simulink model "DataCenterStability"  (R2025b)
settings: Solver=daessc  StartTime=0  StopTime=7  FixedStep=5e-5  MaxStep=0.001  RelTol=1e-3
PostLoadFcn:
  | DataCenterParamScan
InitFcn:
  | opFile_ = fullfile(fileparts(which('DataCenterStability')), 'DataCenterStability_SteadyStateOP.mat');
  | if isfile(opFile_)
  |     tmp_ = load(opFile_, 'op');
  |     assignin('base', 'ssOP__', tmp_.op);
  | end
  | warning('off','physmod:common:mf:system:xform:DelayUnsupportedWithOperatingPoint');
  | warning('off','physmod:common:mf:system:xform:TimeUnsupportedWithOperatingPoint');
values from neighbouring files (symbols this model uses):
  baseVoltageDC = ups.Vdc    [DataCenterParamScan.m]
  bessConverterEfficiency = ups.DCBus.converterEff    [DataCenterParamScan.m]
  droopGain = ups.DCBus.droop    [DataCenterParamScan.m]
  filterInductance = ups.inverter.filterInductance    [DataCenterParamScan.m]
  filterInductanceAFE = ups.AFE.filterInductance    [DataCenterParamScan.m]
  filterResistance = ups.inverter.filterResistance    [DataCenterParamScan.m]
  filterResistanceAFE = ups.AFE.filterResistance    [DataCenterParamScan.m]
  frequency = ups.frequency    [DataCenterParamScan.m]
  G1 = 1    [DataCenterParamScan.m]
  G2 = 0    [DataCenterParamScan.m]
  iBatt = ups.batt.iRated    [DataCenterParamScan.m]
  initialMode = ups.batt.initialMode    [DataCenterParamScan.m]
  invKiId = ups.inverter.kiId    [DataCenterParamScan.m]
  invKiVd = ups.inverter.kiVd    [DataCenterParamScan.m]
  invKpId = ups.inverter.kpId    [DataCenterParamScan.m]
  invKpVd = ups.inverter.kpVd    [DataCenterParamScan.m]
  kpDC = ups.DCBus.kpDC    [DataCenterParamScan.m]
  N_pfc = round(N_total * [1/3, 1/3, 1/3])    [DataCenterParamScan.m]    (also in StabilityStudy.m = cfg.Topology.N_pfc)
  plantRating = ups.rating    [DataCenterParamScan.m]
  powerTau = 0.005    [DataCenterParamScan.m]
  rampRate = ups.batt.rampRate    [DataCenterParamScan.m]
  scan = obj.Cfg.GNC    [GNCAnalyzer.m]
  Ts = 5e-5    (= 5e-05)    [DataCenterParamScan.m]
  Vac = ups.Vac    [DataCenterParamScan.m]
  vBattMax = ups.batt.VMax    [DataCenterParamScan.m]
  vBattNom = ups.batt.Vnom    [DataCenterParamScan.m]
  vDCThreshold = ups.DCBus.VThreshold    [DataCenterParamScan.m]
  vGridMin = ups.DCBus.gridThreshold    [DataCenterParamScan.m]
undefined symbols (not defined in the file or in its folder): ctLimitDelayTime, DiscIntNeverNeededParam, ee_sli_rtmsupport, gcbh, itTray, pfc, serverTray, ups
libraries: fl_lib x77, nesl_utility x35, ee_lib x30, simulink x17, eeGeneralControl x14, datacenter_lib x12, eeTransforms x7, slpidlib x4, nesl_utility_internal x4, simulink_extras x3, datacenterCompositeLib x2, eePowerMeasurement x2
(part 5 of 5)

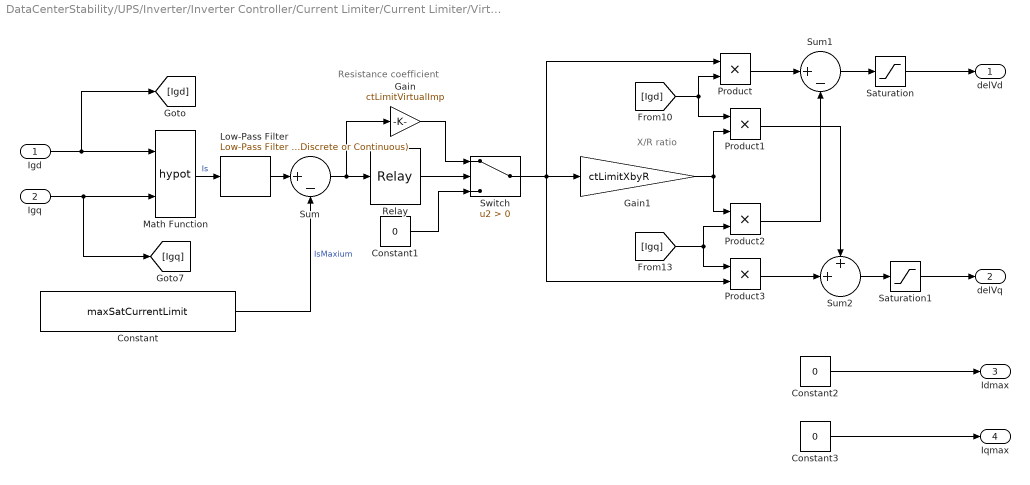
== system DataCenterStability/UPS/Inverter/Inverter Controller/Current Limiter/Current Limiter/Virtual Impedance ==
  note: X/R ratio
  note: Resistance coefficient
  Igd : Inport
  Igq : Inport  Port=2
  Constant : Constant  Value=maxSatCurrentLimit
  Constant1 : Constant  Value=0
  Constant2 : Constant  Value=0
  Constant3 : Constant  Value=0
  Gain : Gain  Gain=ctLimitVirtualImp
  Gain1 : Gain  Gain=ctLimitXbyR
  Low-Pass Filter : eeGeneralControl/Low-Pass Filter (Discrete or Continuous)  K=1  T=1e-3  B=inf  A=-inf  init_option=Inherited from block input  x0=0  Ts=-1
  Math Function : Math  Operator=hypot
  Product{,1..3} (4 alike) : Product
  Relay : Relay  OnSwitchValue=0.01  OffSwitchValue=-0.05
  Saturation : Saturate  UpperLimit=1  LowerLimit=-1
  Saturation1 : Saturate  UpperLimit=1  LowerLimit=-1
  Sum : Sum  Inputs=|+-
  Sum1 : Sum  Inputs=|+-
  Sum2 : Sum  Inputs=++|
  Switch : Switch  Criteria=u2 > Threshold  SaturateOnIntegerOverflow=off  InputSameDT=off
  delVd : Outport
  delVq : Outport  Port=2
  Idmax : Outport  Port=3
  Iqmax : Outport  Port=4
  wires:
  Sum/1 -> Gain/1, Relay/1
  Igq/1 -> [Igq], Math Function/2
  Product1/1 -> Sum2/1
  Gain1/1 -> Product1/2, Product2/1
  Sum1/1 -> Saturation/1
  Product/1 -> Sum1/1
  Product2/1 -> Sum1/2
  Constant/1 -> Sum/2  "IsMaxium"
  Math Function/1 -> Low-Pass Filter/1  "Is"
  [Igq] -> Product3/1, Product2/2
  Switch/1 -> Gain1/1, Product3/2, Product/1
  [Igd] -> Product1/1, Product/2
  Constant2/1 -> Idmax/1
  Constant3/1 -> Iqmax/1
  Gain/1 -> Switch/1
  Constant1/1 -> Switch/3
  Igd/1 -> Math Function/1, [Igd]
  Saturation1/1 -> delVq/1
  Relay/1 -> Switch/2
  Saturation/1 -> delVd/1
  Low-Pass Filter/1 -> Sum/1
  Product3/1 -> Sum2/2
  Sum2/1 -> Saturation1/1

== system DataCenterStability/UPS/Inverter/Inverter Controller/VoltageCurrentControl/Controller/Id Current Limiting ==
  Imax : Inport
  Id : Inport  Port=2
  Abs : Abs  SaturateOnIntegerOverflow=off
  Switch : Switch  Criteria=u2 > Threshold  SaturateOnIntegerOverflow=off  InputSameDT=off
  Idref : Outport
  wires:
  Id/1 -> Switch/3
  Abs/1 -> Switch/2
  Imax/1 -> Abs/1, Switch/1
  Switch/1 -> Idref/1

== system DataCenterStability/UPS/Inverter/Inverter Controller/VoltageCurrentControl/Controller/Iq Current Limiting ==
  Imax : Inport
  Iq : Inport  Port=2
  Abs : Abs  SaturateOnIntegerOverflow=off
  Switch : Switch  Criteria=u2 > Threshold  SaturateOnIntegerOverflow=off  InputSameDT=off
  Iqref : Outport
  wires:
  Iq/1 -> Switch/3
  Abs/1 -> Switch/2
  Imax/1 -> Abs/1, Switch/1
  Switch/1 -> Iqref/1

== system DataCenterStability/UPS/Inverter/Inverter Controller/VoltageCurrentControl/Controller/Voltage control ==
  e : Inport
  Discrete-Time Integrator : DiscreteIntegrator  IntegratorMethod=Integration: Backward Euler  SampleTime=voltControlTs  LimitOutput=on  UpperSaturationLimit=VdMaxCt  LowerSaturationLimit=VdMinCt  ICPrevOutput=DiscIntNeverNeededParam  ICPrevScaledInput=DiscIntNeverNeededParam
  Ki : Gain  Gain=VdIGain
  Kp : Gain  Gain=vdPGain
  Limit : Saturate  UpperLimit=VdMaxCt  LowerLimit=VdMinCt
  Scope : Scope  NumInputPorts=2
      settings: ActiveDisplayYMinimum=-1  ActiveDisplayYMaximum=1  DataLoggingVariableName=ScopeData7
  Scope1 : Scope
      settings: ActiveDisplayYMinimum=-3.0269325328896544E+14  ActiveDisplayYMaximum=2.722979055938979E+15  DataLoggingVariableName=ScopeData8
  Sum7 : Sum  Inputs=|++
  u : Outport  VectorParamsAs1DForOutWhenUnconnected=off
  wires:
  e/1 -> Scope1/1, Ki/1, Kp/1
  Sum7/1 -> Limit/1
  Ki/1 -> Discrete-Time Integrator/1
  Limit/1 -> u/1
  Kp/1 -> Scope/1, Sum7/1
  Discrete-Time Integrator/1 -> Scope/2, Sum7/2

== system DataCenterStability/UPS/Inverter/Inverter Controller/VoltageCurrentControl/Controller/Voltage control1 ==
  e : Inport
  Discrete-Time Integrator : DiscreteIntegrator  IntegratorMethod=Integration: Backward Euler  SampleTime=voltControlTs  LimitOutput=on  UpperSaturationLimit=VqMaxCt  LowerSaturationLimit=VqMinCt  ICPrevOutput=DiscIntNeverNeededParam  ICPrevScaledInput=DiscIntNeverNeededParam
  Ki : Gain  Gain=VqIGain
  Kp : Gain  Gain=VqPGain
  Limit : Saturate  UpperLimit=VqMaxCt  LowerLimit=VqMinCt
  Scope : Scope  NumInputPorts=2
      settings: ActiveDisplayYMinimum=-1  ActiveDisplayYMaximum=1  DataLoggingVariableName=ScopeData43
  Sum7 : Sum  Inputs=|++
  u : Outport  VectorParamsAs1DForOutWhenUnconnected=off
  wires:
  Limit/1 -> u/1
  Ki/1 -> Discrete-Time Integrator/1
  Kp/1 -> Scope/1, Sum7/1
  e/1 -> Kp/1, Ki/1
  Sum7/1 -> Limit/1
  Discrete-Time Integrator/1 -> Scope/2, Sum7/2

== system DataCenterStability/UPS/Inverter/Inverter Controller/VoltageCurrentControl/Controller/d-axis current control ==
  e : Inport
  Discrete-Time Integrator : DiscreteIntegrator  IntegratorMethod=Integration: Backward Euler  SampleTime=currentControlTs  LimitOutput=on  UpperSaturationLimit=4  LowerSaturationLimit=-4  ICPrevOutput=DiscIntNeverNeededParam  ICPrevScaledInput=DiscIntNeverNeededParam
  Ki : Gain  Gain=IdIGain
  Kp : Gain  Gain=IdPGain
  Limit : Saturate  UpperLimit=4  LowerLimit=-4
  Sum7 : Sum  Inputs=|++
  u : Outport  VectorParamsAs1DForOutWhenUnconnected=off
  wires:
  Ki/1 -> Discrete-Time Integrator/1
  Limit/1 -> u/1
  Kp/1 -> Sum7/1
  e/1 -> Kp/1, Ki/1
  Sum7/1 -> Limit/1
  Discrete-Time Integrator/1 -> Sum7/2

== system DataCenterStability/UPS/Inverter/Inverter Controller/VoltageCurrentControl/Controller/q-axis current control ==
  e : Inport
  Discrete-Time Integrator : DiscreteIntegrator  IntegratorMethod=Integration: Backward Euler  SampleTime=currentControlTs  LimitOutput=on  UpperSaturationLimit=3  LowerSaturationLimit=-3  ICPrevOutput=DiscIntNeverNeededParam  ICPrevScaledInput=DiscIntNeverNeededParam
  Ki : Gain  Gain=IqIGain
  Kp : Gain  Gain=IqPGain
  Limit : Saturate  UpperLimit=3  LowerLimit=-3
  Sum7 : Sum  Inputs=|++
  u : Outport  VectorParamsAs1DForOutWhenUnconnected=off
  wires:
  Discrete-Time Integrator/1 -> Sum7/2
  Limit/1 -> u/1
  Sum7/1 -> Limit/1
  e/1 -> Ki/1, Kp/1
  Kp/1 -> Sum7/1
  Ki/1 -> Discrete-Time Integrator/1

== system DataCenterStability/UPS/Rectifier/PFC Rectifier Controller/DC Voltage Controller and Current Reference/Voltage Controller/Voltage control ==
  e : Inport
  Reset : Inport  Port=2
  Discrete-Time Integrator : DiscreteIntegrator  IntegratorMethod=Integration: Backward Euler  ExternalReset=falling  SampleTime=ups.sampleTime  LimitOutput=on  UpperSaturationLimit=2  LowerSaturationLimit=-2  ICPrevOutput=DiscIntNeverNeededParam  ICPrevScaledInput=DiscIntNeverNeededParam
  Ki : Gain  Gain=KiVoltage
  Kp : Gain  Gain=KpVoltage
  Sum7 : Sum  Inputs=|++
  u : Outport  VectorParamsAs1DForOutWhenUnconnected=off
  wires:
  e/1 -> Ki/1, Kp/1
  Ki/1 -> Discrete-Time Integrator/1
  Sum7/1 -> u/1
  Kp/1 -> Sum7/1
  Discrete-Time Integrator/1 -> Sum7/2
  Reset/1 -> Discrete-Time Integrator/2

== system DataCenterStability/UPS/Inverter/Inverter Controller/Current Limiter/Current Limiter/Current Saturation/Compare ==
  u : Inport
  AND : Logic  IconShape=distinctive  AllPortsSameDT=off  OutDataTypeStr=boolean
  Compare To Constant : simulink/Logic and Bit Operations/Compare To Constant  relop=>  const=ctLimitDelayTime  OutDataTypeStr=boolean
  Compare To Zero : simulink/Logic and Bit Operations/Compare To Zero  relop=<=  OutDataTypeStr=boolean
  Data Type Conversion : DataTypeConversion  SaturateOnIntegerOverflow=off  RndMeth=Floor
  Data Type Conversion1 : DataTypeConversion  SaturateOnIntegerOverflow=off  RndMeth=Floor
  Discrete-Time Integrator : DiscreteIntegrator  IntegratorMethod=Integration: Backward Euler  ExternalReset=level  SampleTime=currentControlTs  LimitOutput=on  UpperSaturationLimit=ctLimitDelayTime*2  LowerSaturationLimit=0  ICPrevOutput=DiscIntNeverNeededParam  ICPrevScaledInput=DiscIntNeverNeededParam
  Out1 : Outport
  wires:
  AND/1 -> Data Type Conversion/1
  Compare To Zero/1 -> Data Type Conversion1/1
  Compare To Constant/1 -> AND/2
  u/1 -> Compare To Zero/1
  Discrete-Time Integrator/1 -> Compare To Constant/1
  Data Type Conversion/1 -> Out1/1
  Data Type Conversion1/1 -> Discrete-Time Integrator/2, Discrete-Time Integrator/1, AND/1

== system DataCenterStability/UPS/Inverter/Inverter Controller/Current Limiter/Current Limiter/Current Saturation/If Action Subsystem ==
  Is : Inport
  Isd : Inport  Port=2
  Isq : Inport  Port=3
  Action Port : ActionPort
  Constant : Constant  Value=maxSatCurrentLimit
  Divide : Product  Inputs=*/
  Product : Product
  Product1 : Product
  Idmax : Outport
  Iqmax : Outport  Port=2
  wires:
  Constant/1 -> Divide/1
  Is/1 -> Divide/2
  Divide/1 -> Product1/2, Product/1
  Isd/1 -> Product1/1
  Isq/1 -> Product/2
  Product1/1 -> Idmax/1
  Product/1 -> Iqmax/1

== system DataCenterStability/UPS/Inverter/Inverter Controller/Current Limiter/Current Limiter/Current Saturation/If Action Subsystem1 ==
  Action Port : ActionPort
  Constant3 : Constant  Value=0
  Constant4 : Constant  Value=0
  Idmax : Outport
  Iqmax : Outport  Port=2
  wires:
  Constant4/1 -> Iqmax/1
  Constant3/1 -> Idmax/1

== stateflow chart DataCenterStability/UPS/DC-Link/BESS/DC-DC Converter Controller/Mode Control/BMS ==
  state Discharge
    entry :
    mode = 4;
    if VPCC <= 0.1
    droopMode = 0;
    else
    droopMode = 1;
    end
    during:
    if VPCC <= 0.1
    droopMode = 0;
    else
    droopMode = 1;
    end
    vOut = Vdc/VdcRated;
    iRef = 0;
    flagCVChrg =  breakerStatus <=0 && VBatt >= VMaxBatt && abs(iBatt) < iBattTh && VPCC >= 0.8;
    flagCCChrg = breakerStatus <=0 && VBatt <= VMaxBatt && abs(iBatt) < iBattTh && VPCC >= 0.8;
  state Stand_by
    entry :
    mode = initialMode;
  state Float_Charging
    entry :
    mode = 3;
    during:
    vOut = VMaxBatt/VBattNom;
    iRef = 0;
    flagFloatDchrg = iPFC <= iThreshold || Vdc <= VMaxDC...
    || VPCC <= vThreshold;
  state Constant_Voltage_Charging
    entry :
    mode = 2;
    during:
    vOut = 1;
    iRef = 0;
    flagCVDchrg = (iPFC <= iThreshold || Vdc <= VMaxDC) || VPCC <= vThreshold
  state Constant_Current_Charging
    entry :
    mode = 1;
    during:
    vOut = 1;
    iRef = iCharg;
    flagCCDchrg = (iPFC <= iThreshold || Vdc <= VMaxDC) || VPCC <= vThreshold;
  (default) -> Stand_by
  Stand_by -> (junction 521) : [after(1,sec)]
  Float_Charging -> (junction 571) : [duration(flagFloatDchrg, sec) > 0.01]
  (junction 521) -> Discharge [order 1] : [mode == 4]
  (junction 521) -> Float_Charging [order 2] : [SOC >= 0.98]
  (junction 571) -> (junction 573)
  (junction 521) -> (junction 522) [order 3]
  (junction 577) -> Discharge
  (junction 575) -> (junction 577)
  (junction 566) -> Discharge
  Discharge -> (junction 524) [order 2]
  Discharge -> (junction 523) [order 1]
  (junction 580) -> Discharge
  Constant_Voltage_Charging -> Float_Charging [order 1] : [SOC >= 0.98]
  Constant_Voltage_Charging -> (junction 546) [order 2] : [duration(flagCVDchrg, sec) > 0.01]
  (junction 546) -> (junction 548)
  (junction 522) -> Constant_Voltage_Charging [order 1] : [SOC <= 0.98 && VBatt >=VMaxBatt]
  (junction 525) -> Constant_Voltage_Charging
  (junction 522) -> (junction 531) [order 2]
  (junction 527) -> (junction 525) : [duration(flagCVChrg >0 ,sec)>0.01]
  Constant_Current_Charging -> Constant_Voltage_Charging [order 1] : [VBatt >= VMaxBatt]
  (junction 531) -> Constant_Current_Charging : [SOC <=0.98 && VBatt <= VMaxBatt]
  Constant_Current_Charging -> (junction 580) [order 2] : [duration(flagCCDchrg,sec)>0.5]
  (junction 523) -> Constant_Current_Charging : [duration(flagCCChrg ,sec) > 0.5]
  (junction 524) -> (junction 527)
  (junction 548) -> (junction 566)
  (junction 573) -> (junction 575)
  data: iPFC input double; iThreshold parameter double; Vdc input double; VMaxBatt parameter double; VMaxDC parameter double; mode output double; VBatt input double =400; SOC input double; initialMode parameter; breakerStatus input; VBattNom parameter; vThreshold parameter; VPCC input; iCharg input; iRef output; vOut output; VdcRated parameter; flagCVChrg local boolean =0; flagCCDchrg local boolean =0; flagCVDchrg local boolean =0; flagFloatDchrg local boolean =0; flagCCChrg local boolean =0; iBatt input; iBattTh parameter; droopMode output
